simulink library "Brake_System_Completion_of_Recuperation"  (R2018b)
settings: Solver=VariableStepAuto  StartTime=0.0  StopTime=10.0  RelTol=1e-3
settings Model: Creator=Alexander Koch  LastModifiedBy=ga69qig
settings SFSimCC: SimUseLocalCustomCode=off
settings RTWCC: RTWUseLocalCustomCode=off
settings CodeAppCC: StateflowObjectComments=on

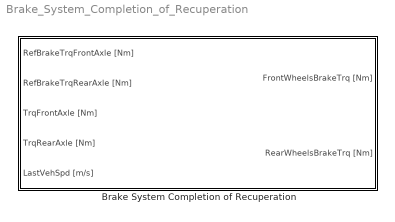
== system Brake_System_Completion_of_Recuperation ==
  Brake System Completion of Recuperation : Subsystem  mask(SB){LocalSampleTime=-1}
      mask prompts: LocalSampleTime "Local System Sample-Time [s]"
      mask help:
      | <Author> Alexander Koch, Benedikt Danquah based on Stefan Müller [1], Stephan Rohr [2]  </Author>
      | <Datum> 21/03/2017 </Datum>
      |
      | <Description>
      | Calculates the required braking torque for the front and the rear wheel that has to be added through the brakes and is not applied by the recuperation of the motor.
      | </Description>
      mask init:
      | GlobalSampleTime = CalcGlobalSampleTime(LocalSampleTime)
      mask Help:
      | <Parameters>
      | Local System Sample-Time [s]
      | 	<Min> GlobalSampleTime </Min>
      | Global Sample-Time [s]
      | </Parameters>
      | 
      | <Inputs>
      | RefBrakeTrqFrontAxle [Nm]
      | 	<sign orientation> [+] braking </sign orientation>
      | RefBrakeTrqRearAxle [Nm]
      | 	<sign orientation> [+] braking </sign orientation>
      | TrqFrontAxle [Nm]
      | 	<sign orientation> [-] recuperation </sign orientation>
      | TrqRearAxle [Nm]
      | 	<sign orientation> [-] recuperation </sign orientation>
      | LastVehSpd [m/s]
      | </Inputs>
      | 
      | <Outputs>
      | FrontWheelsBrakeTrq [Nm]
      | 	<Max> 0 </Max>
      | 	<sign orientation> [+] braking </sign orientation>
      | RearWheelsBrakeTrq [Nm]
      | 	<Max> 0 </Max>
      | 	<sign orientation> [+] braking </sign orientation>
      | </Outputs>
      | 
      | <Sources>
      | [1] S. Mueller, S. Rohr, W. Schmid, and M. Lienkamp, “Analysing the Influence of Driver Behaviour and Tuning Measures on Battery Aging and Residual Value of Electric Vehicles,” in Proc. EVS30 Symposium, Stuttgart, 2017, pp. 1–12.
      | [2] S. Rohr, “Technisch-wirtschaftliche Analyse des Zweitnutzungs- potentials von Lithium-Ionen-Traktionsbatterien,” Dissertation, Institute of Automotive Technology, Technical University Munich, Munich, 2018.
      | </Sources>
      mask TypeOptions LocalSampleTime: RefBrakeTrqFrontAxle [Nm]/SampleTime | RefBrakeTrqRearAxle [Nm]/SampleTime | TrqFrontAxle [Nm]/SampleTime | TrqRearAxle [Nm]/SampleTime | LastVehSpd [m//s]/SampleTime
      mask DialogControl DescGroupVar1 Prompt: Documentation:
      mask DialogControl Control2 Prompt: %<MaskHelp>
      mask DialogControl Container3 Prompt: Sample Time
      mask Display:
      | [picturexpos,pictureypos,picturewidth,pictureheight] = ...
      |     CalcBlockPicturePosition(gcb,1,0.01,0.1,100,100); % calculating picture position depending on Block size and minimum margin size
      | image('Brake_System_Completion_of_Recuperation.svg',[picturexpos pictureypos picturewidth pictureheight]) % plot picture to block

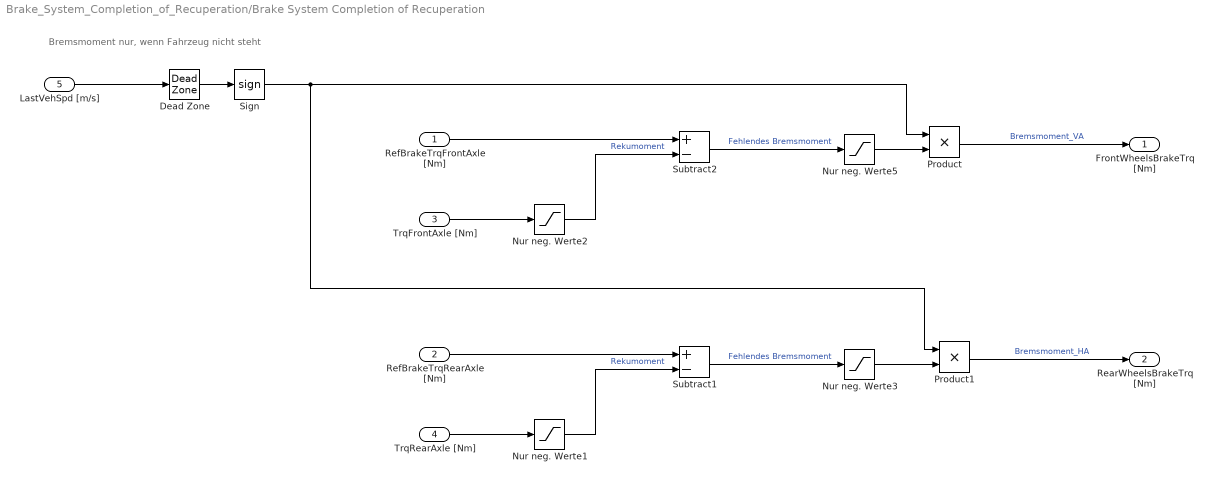
== system Brake_System_Completion_of_Recuperation/Brake System Completion of Recuperation ==
  note: Bremsmoment nur, wenn Fahrzeug nicht steht
  RefBrakeTrqFrontAxle [Nm] : Inport  SampleTime=LocalSampleTime
  RefBrakeTrqRearAxle [Nm] : Inport  Port=2  SampleTime=LocalSampleTime
  TrqFrontAxle [Nm] : Inport  Port=3  SampleTime=LocalSampleTime
  TrqRearAxle [Nm] : Inport  Port=4  SampleTime=LocalSampleTime
  LastVehSpd [m/s] : Inport  Port=5  SampleTime=LocalSampleTime
  Dead Zone : DeadZone  LowerValue=-0.2  UpperValue=0.2  SaturateOnIntegerOverflow=on
  Nur neg. Werte{1..3,5} (4 alike) : Saturate  UpperLimit=0  LowerLimit=-inf
  Product : Product
  Product1 : Product
  Sign : Signum
  Subtract1 : Sum  Inputs=+-
  Subtract2 : Sum  Inputs=+-
  FrontWheelsBrakeTrq [Nm] : Outport  SampleTime=GlobalSampleTime
  RearWheelsBrakeTrq [Nm] : Outport  Port=2  SampleTime=GlobalSampleTime
  wires:
  Subtract1/1 -> Nur neg. Werte3/1  "Fehlendes Bremsmoment"
  Product1/1 -> RearWheelsBrakeTrq [Nm]/1  "Bremsmoment_HA"
  TrqFrontAxle [Nm]/1 -> Nur neg. Werte2/1
  Subtract2/1 -> Nur neg. Werte5/1  "Fehlendes Bremsmoment"
  Sign/1 -> Product1/1, Product/1
  LastVehSpd [m/s]/1 -> Dead Zone/1
  RefBrakeTrqRearAxle [Nm]/1 -> Subtract1/1
  RefBrakeTrqFrontAxle [Nm]/1 -> Subtract2/1
  Product/1 -> FrontWheelsBrakeTrq [Nm]/1  "Bremsmoment_VA"
  Nur neg. Werte3/1 -> Product1/2
  Nur neg. Werte5/1 -> Product/2
  TrqRearAxle [Nm]/1 -> Nur neg. Werte1/1
  Nur neg. Werte2/1 -> Subtract2/2  "Rekumoment"
  Nur neg. Werte1/1 -> Subtract1/2  "Rekumoment"
  Dead Zone/1 -> Sign/1
